simulink model "suspension_sys_main"  (Simulink 7.0)
settings: Solver=ode45  StartTime=0.0  StopTime=10.0  RelTol=1e-3
model workspace (MAT data in the model file):
  M1 = 2500
  M2 = 320
  k1 = 80000
  k2 = 500000
  b1 = 350
  b2 = 15020
  Mse = 90
  Ms = 250
  Mu = 40
  bs = 2000
  bse = 3000
  Kt = 125000
  Ks = 28000
  Kse = 8000
  Zr : num (value not decoded)
values from neighbouring files (symbols this model uses):
  bs = 2000    [suspension_sys_MATLAB.m]    (also in suspensiondata.mat)
  bse = 3000    [suspension_sys_MATLAB.m]    (also in suspensiondata.mat)
  Ks = 28000    [suspension_sys_MATLAB.m]    (also in suspensiondata.mat)
  Kse = 8000    [suspension_sys_MATLAB.m]    (also in suspensiondata.mat)
  Kt = 125000    [suspension_sys_MATLAB.m]    (also in suspensiondata.mat)
  Ms = 250    [suspension_sys_MATLAB.m]    (also in suspensiondata.mat)
  Mse = 90    [suspension_sys_MATLAB.m]    (also in suspensiondata.mat)
  Mu = 40    [suspension_sys_MATLAB.m]    (also in suspensiondata.mat)
  Zr = 0.2    [suspension_sys_MATLAB.m]    (also in suspensiondata.mat)
settings Model: Creator=kiran.jacob  LastModifiedBy=kiran.jacob

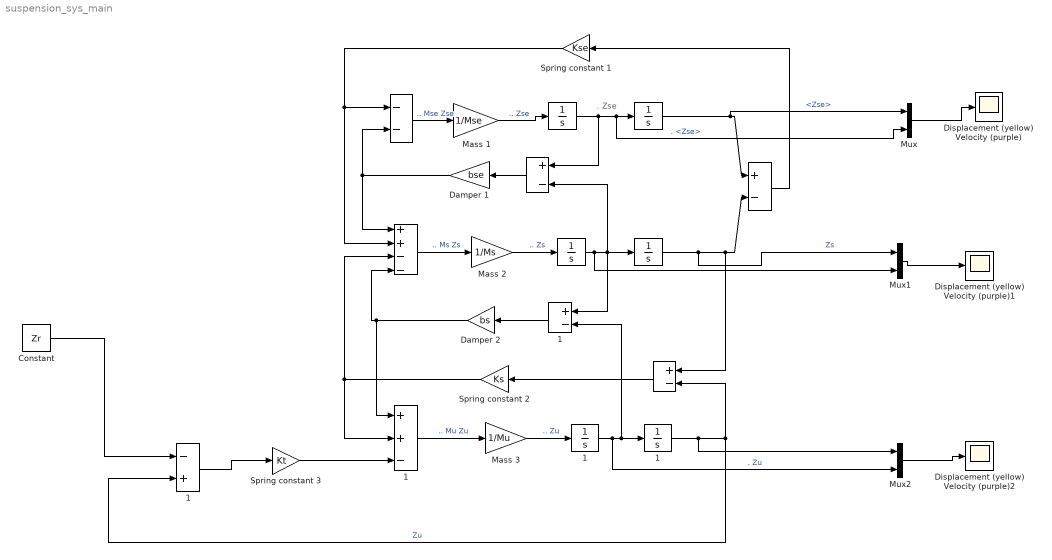
== system suspension_sys_main ==
  note: .
      | Zse
  " " : Integrator
  "  " : Sum  Inputs=+-  OutDataType=sfix(16)  OutScaling=2^-10
  "     " : Integrator
  "      " : Sum  Inputs=++--  OutDataType=sfix(16)  OutScaling=2^-10
  "       " : Sum  Inputs=--  OutDataType=sfix(16)  OutScaling=2^-10
  "        " : Sum  Orientation=left  Inputs=+-  OutDataType=sfix(16)  OutScaling=2^-10
  "         " : Integrator
  "          " : Integrator
  "             " : Sum  Orientation=left  Inputs=+-  OutDataType=sfix(16)  OutScaling=2^-10
  "             1" : Sum  Orientation=left  Inputs=+-  OutDataType=sfix(16)  OutScaling=2^-10
  "          1" : Integrator
  "         1" : Integrator
  "       1" : Sum  Inputs=-+  OutDataType=sfix(16)  OutScaling=2^-10
  "      1" : Sum  Inputs=++-  OutDataType=sfix(16)  OutScaling=2^-10
  Constant : Constant  Value=Zr  OutDataType=sfix(16)  OutScaling=2^0
  Damper 1 : Gain  Orientation=left  Gain=bse  ParameterDataType=sfix(16)  ParameterScaling=2^0  OutDataType=sfix(16)  OutScaling=2^0
  Damper 2 : Gain  Orientation=left  Gain=bs  ParameterDataType=sfix(16)  ParameterScaling=2^0  OutDataType=sfix(16)  OutScaling=2^0
  Displacement (yellow) Velocity (purple) : Scope
      settings: TimeRange=10  YMin=-1  YMax=1.5
  Displacement (yellow) Velocity (purple)1 : Scope
      settings: TimeRange=10  YMin=-1  YMax=1.5
  Displacement (yellow) Velocity (purple)2 : Scope
      settings: TimeRange=10  YMin=-2  YMax=7  SaveName=ScopeData2
  Mass 1 : Gain  Gain=1/Mse  ParameterDataType=sfix(16)  ParameterScaling=2^0  OutDataType=sfix(16)  OutScaling=2^0
  Mass 2 : Gain  Gain=1/Ms  ParameterDataType=sfix(16)  ParameterScaling=2^0  OutDataType=sfix(16)  OutScaling=2^0
  Mass 3 : Gain  Gain=1/Mu  ParameterDataType=sfix(16)  ParameterScaling=2^0  OutDataType=sfix(16)  OutScaling=2^0
  Mux : Mux  Inputs=2
  Mux1 : Mux  Inputs=2
  Mux2 : Mux  Inputs=2
  Spring constant 1 : Gain  Orientation=left  Gain=Kse  ParameterDataType=sfix(16)  ParameterScaling=2^0  OutDataType=sfix(16)  OutScaling=2^0
  Spring constant 2 : Gain  Orientation=left  Gain=Ks  ParameterDataType=sfix(16)  ParameterScaling=2^0  OutDataType=sfix(16)  OutScaling=2^0
  Spring constant 3 : Gain  Gain=Kt  ParameterDataType=sfix(16)  ParameterScaling=2^0  OutDataType=sfix(16)  OutScaling=2^0
  wires:
  " "/1 -> "        "/1, "     "/1, Mux/2  ". <Zse>"
  "         "/1 -> "        "/2, "          "/1, "             1"/1, Mux1/2
  Mass 1/1 -> " "/1  ".. Zse"
  Mass 2/1 -> "         "/1  ".. Zs"
  "       "/1 -> Mass 1/1  ".. Mse Zse"
  "      "/1 -> Mass 2/1  ".. Ms Zs"
  "     "/1 -> "  "/1, Mux/1  "<Zse>"
  "          "/1 -> "  "/2, "             "/1, Mux1/1  "Zs"
  "  "/1 -> Spring constant 1/1
  Spring constant 1/1 -> "      "/2, "       "/1
  "        "/1 -> Damper 1/1
  Damper 1/1 -> "      "/1, "       "/2
  "      1"/1 -> Mass 3/1  ".. Mu Zu"
  Mass 3/1 -> "         1"/1  ".. Zu"
  "         1"/1 -> "          1"/1, "             1"/2, Mux2/2  ". Zu"
  "          1"/1 -> "             "/2, "       1"/2, Mux2/1  "Zu"
  "             "/1 -> Spring constant 2/1
  "             1"/1 -> Damper 2/1
  Damper 2/1 -> "      "/4, "      1"/1
  Spring constant 2/1 -> "      "/3, "      1"/2
  Spring constant 3/1 -> "      1"/3
  Constant/1 -> "       1"/1
  "       1"/1 -> Spring constant 3/1
  Mux/1 -> Displacement (yellow) Velocity (purple)/1
  Mux1/1 -> Displacement (yellow) Velocity (purple)1/1
  Mux2/1 -> Displacement (yellow) Velocity (purple)2/1
